simulink model "simulink_implementation"  (R2019b)
settings: Solver=FixedStepDiscrete  StartTime=0.0  StopTime=timetorun  RelTol=1e-3
values from neighbouring files (symbols this model uses):
  buffer_ratio = 22    [workspace.mat]
  dsp_slices = 120    [workspace.mat]
  sample_rate = 3.84615384615e-10    [workspace.mat]
  v_in = [0.247432525758 0.0871400770001 0.120692528926 0.279654863041 0.499712336025 0.162396807443 0.157858677754 0.542160721462 0.0975919889693 0.172516993327 0.21706163112 0.391132018305 ... (26000 elements, 1x26000)]    [workspace.mat]
libraries: hdlsllib x2, dspsrcs4 x2
settings Model: DataTypeOverride=Off  Creator=ian  LastModifiedBy=ian
settings DataIOCC: LimitDataPoints=on  SaveOutput=off  SaveTime=off
settings OptimizationCC: BlockReduction=off  ConditionallyExecuteInputs=off  DefaultParameterBehavior=Inlined  LifeSpan=inf
settings DebuggingCC: SignalRangeChecking=warning  AlgebraicLoopMsg=error  SingleTaskRateTransMsg=error  AllowSymbolicDim=off  StrictBusMsg=ErrorOnBusTreatedAsVector  SFUnexpectedBacktrackingDiag=warning  SFNoUnconditionalDefaultTransitionDiag=warning  SFExecutionAtInitializationDiag=none  ArithmeticOperatorsInVariantConditions=warning
settings HardwareCC: ProdBitPerPointer=32  ProdBitPerSizeT=32  ProdBitPerPtrDiffT=32  ProdLargestAtomicFloat=None  ProdIntDivRoundTo=Undefined  ProdEndianess=Unspecified  ProdWordSize=32  ProdHWDeviceType=ASIC/FPGA->ASIC/FPGA  TargetBitPerPointer=64  TargetBitPerSizeT=64  TargetBitPerPtrDiffT=64  TargetLongLongMode=on  TargetIntDivRoundTo=Zero  TargetEndianess=LittleEndian  TargetWordSize=64  TargetHWDeviceType=Custom Processor->MATLAB Host Computer  ProdEqTarget=off
settings SFSimCC: SimUseLocalCustomCode=off  CustomCodeUndefinedFunction=UseInterfaceOnly
settings RTWCC: RTWUseLocalCustomCode=off
settings CodeAppCC: StateflowObjectComments=on
settings GRTTargetCC: TargetLangStandard=C89/C90 (ANSI)  GeneratePreprocessorConditionals=Disable all
settings ConfigComp: CovScope=ReferencedModels  CovMetricSettings=dw  CovHtmlReporting=on  CovSaveCumulativeToWorkspaceVar=on  CovSaveSingleToWorkspaceVar=on  CovExternalEMLEnable=off  CovSFcnEnable=off

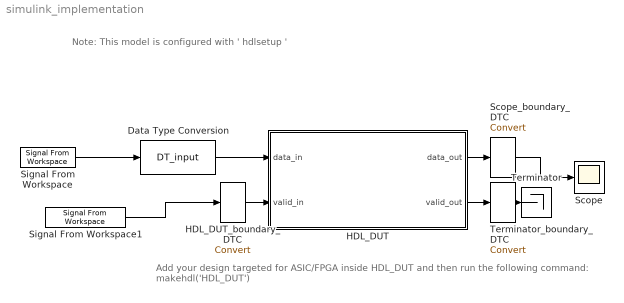
== system simulink_implementation ==
  note: Note: This model is configured with ' hdlsetup '
  note: Add your design targeted for ASIC/FPGA inside HDL_DUT and then run the following command:
      | makehdl('HDL_DUT')
  Data Type Conversion : DataTypeConversion  OutDataTypeStr=DT_input
  HDL_DUT : Subsystem
  HDL_DUT_boundary_DTC : DataTypeConversion  SaturateOnIntegerOverflow=on  RndMeth=Zero
  Scope : Scope
  Scope_boundary_DTC : DataTypeConversion  SaturateOnIntegerOverflow=on  RndMeth=Zero
  Signal From Workspace : dspsrcs4/Signal From Workspace  X=v_in  Ts=sample_rate  nsamps=dsp_slices  OutputAfterFinalValue=Setting to zero  ignoreOrWarnInputAndFrameLengths=off  OutputFrames=off
  Signal From Workspace1 : dspsrcs4/Signal From Workspace  X=true(size(v_in))  Ts=sample_rate  nsamps=1  OutputAfterFinalValue=Setting to zero  ignoreOrWarnInputAndFrameLengths=off  OutputFrames=off
  Terminator : Terminator
  Terminator_boundary_DTC : DataTypeConversion  SaturateOnIntegerOverflow=on  RndMeth=Zero
  wires:
  Signal From Workspace/1 -> Data Type Conversion/1
  Data Type Conversion/1 -> HDL_DUT/1(data_in)
  Signal From Workspace1/1 -> HDL_DUT_boundary_DTC/1
  HDL_DUT_boundary_DTC/1 -> HDL_DUT/2(valid_in)
  HDL_DUT/1(data_out) -> Scope_boundary_DTC/1
  Scope_boundary_DTC/1 -> Scope/1
  HDL_DUT/2(valid_out) -> Terminator_boundary_DTC/1
  Terminator_boundary_DTC/1 -> Terminator/1

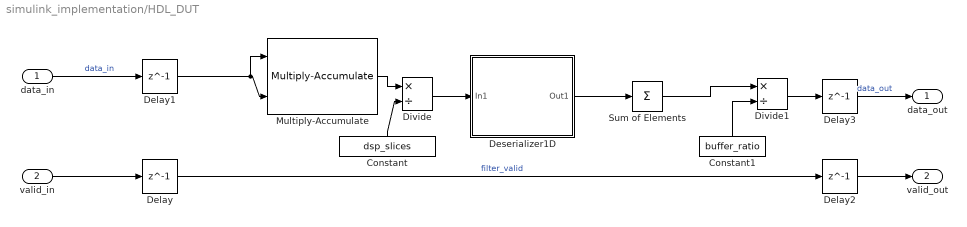
== system simulink_implementation/HDL_DUT ==
  data_in : Inport
  valid_in : Inport  Port=2
  Constant : Constant  Value=dsp_slices  SampleTime=-1
  Constant1 : Constant  Value=buffer_ratio  SampleTime=-1
  Delay{,1..3} (4 alike) : Delay  DelayLength=1
  Deserializer1D : Subsystem  Tag=DecoupledSystem
  Divide : Product  Inputs=*/  SaturateOnIntegerOverflow=on  RndMeth=Zero
  Divide1 : Product  Inputs=*/
  Multiply-Accumulate : hdlsllib/HDL Operations/Multiply-Accumulate  opMode=Vector  initValueSetting=Dialog  initValue=0  initValueSetting2=Dialog  initValue2=0  initValueSetting3=Dialog  initValue3=0  num_samples=5  RndMeth=Nearest  RndMeth2=Floor  RndMeth3=Floor  datatype2=Inherit: Inherit via back propagation  datatype3=fixdt(1,16,0)  validOut=on  endInandOut=on  startOut=on  countOut=on  dim=-1  DoSatur=off  parallel=off
      settings: SourceProductName=Simulink  SourceProductBaseCode=SL
  Sum of Elements : Sum  Inputs=+
  data_out : Outport  VectorParamsAs1DForOutWhenUnconnected=off
  valid_out : Outport  Port=2  VectorParamsAs1DForOutWhenUnconnected=off
  wires:
  data_in/1 -> Delay1/1  "data_in"
  Multiply-Accumulate/1 -> Divide/1
  Constant/1 -> Divide/2
  Divide/1 -> Deserializer1D/1(In1)
  Deserializer1D/1(Out1) -> Sum of Elements/1
  Divide1/1 -> Delay3/1
  Sum of Elements/1 -> Divide1/1
  Constant1/1 -> Divide1/2
  valid_in/1 -> Delay/1
  Delay1/1 -> Multiply-Accumulate/1, Multiply-Accumulate/2
  Delay/1 -> Delay2/1  "filter_valid"
  Delay3/1 -> data_out/1  "data_out"
  Delay2/1 -> valid_out/1

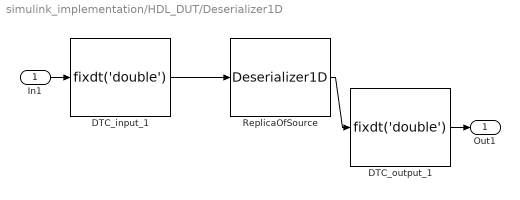
== system simulink_implementation/HDL_DUT/Deserializer1D ==
  In1 : Inport  LockScale=on
  DTC_input_1 : DataTypeConversion  OutDataTypeStr=fixdt('double')  RndMeth=Nearest  LockScale=on
  DTC_output_1 : DataTypeConversion  OutDataTypeStr=fixdt('double')
  ReplicaOfSource : hdlsllib/HDL Operations/Deserializer1D  Ratio=buffer_ratio  IdleCycles=0  InitialCondition=0  startIn=off  validIn=off  validOut=off  inputDataDimensions=-1  inputSampleTime=-1  inputSignalType=auto
      settings: SourceProductName=Simulink  SourceProductBaseCode=SL
  Out1 : Outport  LockScale=on
  wires:
  DTC_output_1/1 -> Out1/1
  ReplicaOfSource/1 -> DTC_output_1/1
  DTC_input_1/1 -> ReplicaOfSource/1
  In1/1 -> DTC_input_1/1
